simulink model "example1"  (R2021b)
settings: Solver=FixedStepDiscrete  StartTime=0.0  StopTime=Tges  RelTol=1e-3
values from neighbouring files (symbols this model uses):
  Ts = simout.SimulationMetadata.ModelInfo.SolverInfo.FixedStepSize    [plot_phi.m]
libraries: simulink x1
settings Model: Creator=siegl  LastModifiedBy=siegl

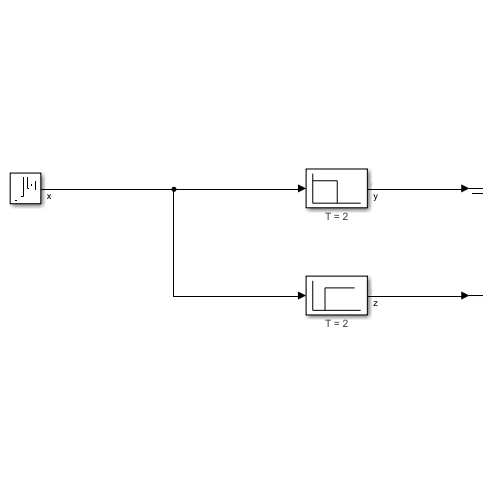
[thumbnail: Simulink's stored preview of the top-level diagram]
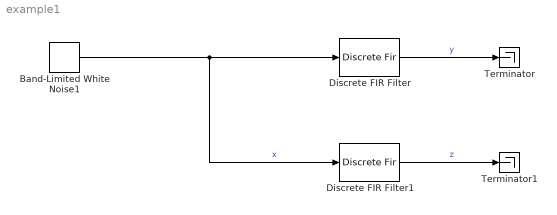
== system example1 ==
  Band-Limited White Noise1 : simulink/Sources/Band-Limited White Noise  Cov=1  Ts=Ts  seed=[23341]
  Discrete FIR Filter : DiscreteFir  Coefficients=ones(1,Tavg/SampleTime)*SampleTime/Tavg  SampleTime=SampleTime  mask{Tavg=2, SampleTime=Ts}
      mask prompts: Tavg "Average Time"; SampleTime "Simulink:blkprm_prompts:AllBlksSampleTime"
      settings: AttributesFormatString=T = %<Tavg>
      mask TypeOptions SampleTime: SampleTime
      mask DialogControl SampleTime Prompt: Sample time (-1 for inherited):
      mask Display:
      | plot([0.1, .9], [.1, .1])
      | plot([0.1, .1], [.1, .9])
      | plot([0.1, .5], [.7, .7])
      | plot([0.5, .5], [.7, .1])
  Discrete FIR Filter1 : DiscreteFir  Coefficients=[zeros(1,Td/SampleTime), 1]  SampleTime=SampleTime  mask{Td=2, SampleTime=Ts}
      mask prompts: Td "Delay Time"; SampleTime "Simulink:blkprm_prompts:AllBlksSampleTime"
      settings: AttributesFormatString=T = %<Td>
      mask TypeOptions SampleTime: SampleTime
      mask DialogControl SampleTime Prompt: Sample time (-1 for inherited):
      mask Display:
      | plot([0.1, .9], [.1, .1])
      | plot([0.1, .1], [.1, .9])
      | plot([0.3, .3], [.7, .1])
      | plot([0.3, .8], [.7, .7])
  Terminator : Terminator
  Terminator1 : Terminator
  wires:
  Band-Limited White Noise1/1 -> Discrete FIR Filter/1, Discrete FIR Filter1/1  "x"
  Discrete FIR Filter1/1 -> Terminator1/1  "z"
  Discrete FIR Filter/1 -> Terminator/1  "y"
